simulink model "dual_quaternion_equation_of_motion_2"  (R2016a)
settings: Solver=VariableStepAuto  StartTime=0.0  StopTime=1000  RelTol=1e-3
InitFcn:
  | addpath('..');
libraries: aerolibconvert2 x6
settings Model: Creator=AkhramovichSA  LastModifiedBy=AkhramovichSA

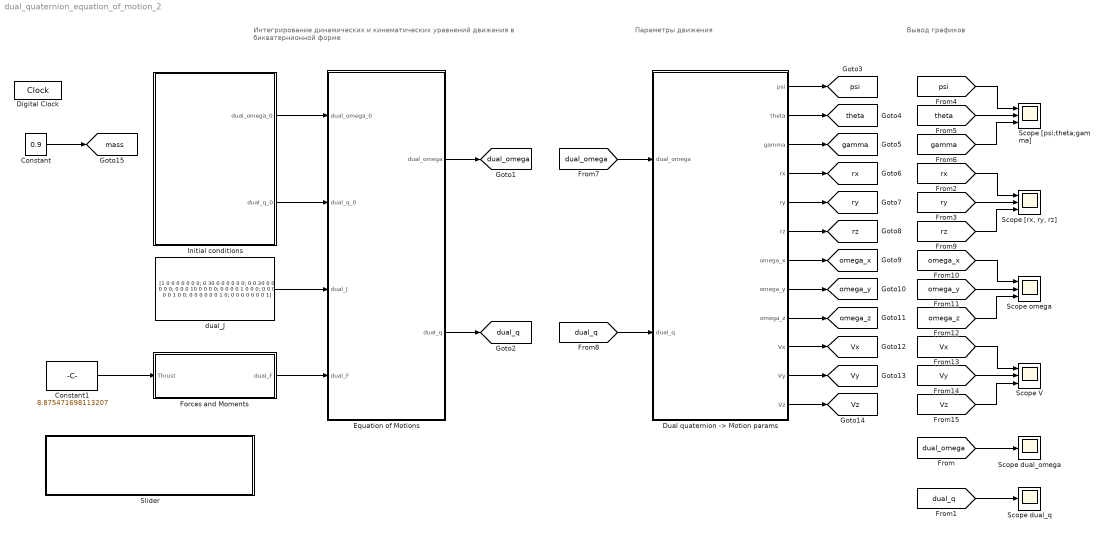
== system dual_quaternion_equation_of_motion_2 ==
  note: Интегрирование динамических и кинематических уравнений движения в бикватернионной форме
  note: Параметры движения
  note: Вывод графиков
  Constant : Constant  Value=0.9
  Constant1 : Constant  Value=8.875471698113207
  Digital Clock : DigitalClock  SampleTime=0.01
  "Dual quaternion -> Motion params" : MATLAB Function  TreatAsAtomicUnit=on
  Equation of Motions : Subsystem
  Forces and Moments : Subsystem
  Initial conditions : Subsystem
  Scope V : Scope  NumInputPorts=3
  Scope [psi;theta;gamma] : Scope  NumInputPorts=3
  "Scope [rx, ry, rz]" : Scope  NumInputPorts=3
  Scope dual_omega : Scope
  Scope dual_q : Scope
  Scope omega : Scope  NumInputPorts=3
  Slider : Subsystem  DialogController=hmiCreateDDGDialog  IsWebBlock=on  mask(MWDashboardBlock){webBlockId=836bae8a-61ff-49e9-8a0b-c22522f8dc87, webBlockType=slider, ShowInLibBrowser=on, ShowInitialText=on, HMISrcModelName=dual_quaternion_equation_of_motion_2}
      mask prompts: webBlockId "WebBlock Id"; webBlockType "WebBlock Type"; HMISrcModelName "Source Model"
      mask Help: helpview([docroot '/mapfiles/simulink.map'], 'hmi_slider')
      mask Display:
      | if strcmp(get_param(bdroot(gcb),'BlockDiagramType'), 'library')
      |     image([(matlabroot) '/toolbox/simulink/hmi/icons/Slider.png']);
      | end
  dual_J : Constant  Value=[1 0 0 0 0 0 0 0; 0 30 0 0 0 0 0 0; 0 0 20 0 0 0 0 0; 0 0 0 10 0 0 0 0; 0 0 0 0 1 0 0 0; 0 0 0 0 0 1 0 0; 0 0 0 0 0 0 1 0; 0 0 0 0 0 0 0 1]  VectorParams1D=off
  tag scope: Vx=global, Vy=global, Vz=global, dual_omega=global, dual_q=global, gamma=global, mass=global, omega_x=global, omega_y=global, omega_z=global, psi=global, rx=global, ry=global, rz=global, theta=global
  wires:
  dual_J/1 -> Equation of Motions/3(dual_J)
  Initial conditions/1(dual_omega_0) -> Equation of Motions/1(dual_omega_0)
  Initial conditions/2(dual_q_0) -> Equation of Motions/2(dual_q_0)
  Forces and Moments/1(dual_F) -> Equation of Motions/4(dual_F)
  Equation of Motions/1(dual_omega) -> [dual_omega]
  [dual_omega] -> Scope dual_omega/1
  Equation of Motions/2(dual_q) -> [dual_q]
  [dual_q] -> Scope dual_q/1
  [psi] -> Scope [psi;theta;gamma]/1
  [theta] -> Scope [psi;theta;gamma]/2
  [gamma] -> Scope [psi;theta;gamma]/3
  [dual_omega] -> "Dual quaternion -> Motion params"/1(dual_omega)
  [dual_q] -> "Dual quaternion -> Motion params"/2(dual_q)
  "Dual quaternion -> Motion params"/1(psi) -> [psi]
  "Dual quaternion -> Motion params"/2(theta) -> [theta]
  "Dual quaternion -> Motion params"/3(gamma) -> [gamma]
  "Dual quaternion -> Motion params"/4(rx) -> [rx]
  "Dual quaternion -> Motion params"/5(ry) -> [ry]
  "Dual quaternion -> Motion params"/6(rz) -> [rz]
  "Dual quaternion -> Motion params"/7(omega_x) -> [omega_x]
  "Dual quaternion -> Motion params"/9(omega_z) -> [omega_z]
  "Dual quaternion -> Motion params"/8(omega_y) -> [omega_y]
  "Dual quaternion -> Motion params"/10(Vx) -> [Vx]
  "Dual quaternion -> Motion params"/11(Vy) -> [Vy]
  "Dual quaternion -> Motion params"/12(Vz) -> [Vz]
  [rx] -> "Scope [rx, ry, rz]"/1
  [ry] -> "Scope [rx, ry, rz]"/2
  [rz] -> "Scope [rx, ry, rz]"/3
  [omega_x] -> Scope omega/1
  [omega_y] -> Scope omega/2
  [omega_z] -> Scope omega/3
  [Vx] -> Scope V/1
  [Vy] -> Scope V/2
  [Vz] -> Scope V/3
  Constant/1 -> [mass]
  Constant1/1 -> Forces and Moments/1(Thrust)

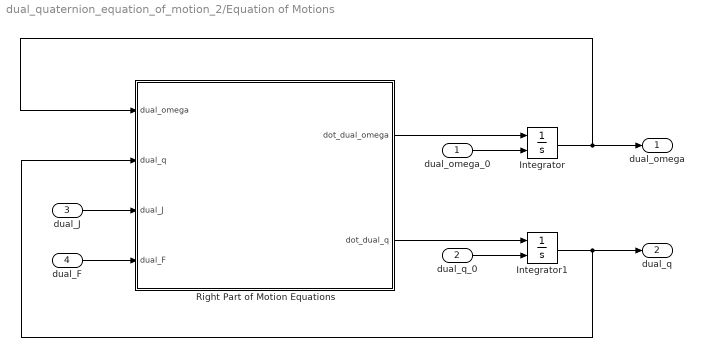
== system dual_quaternion_equation_of_motion_2/Equation of Motions ==
  dual_omega_0 : Inport
  dual_q_0 : Inport  Port=2
  dual_J : Inport  Port=3
  dual_F : Inport  Port=4
  Integrator : Integrator  InitialConditionSource=external
  Integrator1 : Integrator  InitialConditionSource=external
  Right Part of Motion Equations : MATLAB Function  TreatAsAtomicUnit=on
  dual_omega : Outport
  dual_q : Outport  Port=2
  wires:
  Integrator/1 -> dual_omega/1, Right Part of Motion Equations/1(dual_omega)
  dual_omega_0/1 -> Integrator/2
  dual_q_0/1 -> Integrator1/2
  Right Part of Motion Equations/1(dot_dual_omega) -> Integrator/1
  Integrator1/1 -> dual_q/1, Right Part of Motion Equations/2(dual_q)
  Right Part of Motion Equations/2(dot_dual_q) -> Integrator1/1
  dual_F/1 -> Right Part of Motion Equations/4(dual_F)
  dual_J/1 -> Right Part of Motion Equations/3(dual_J)

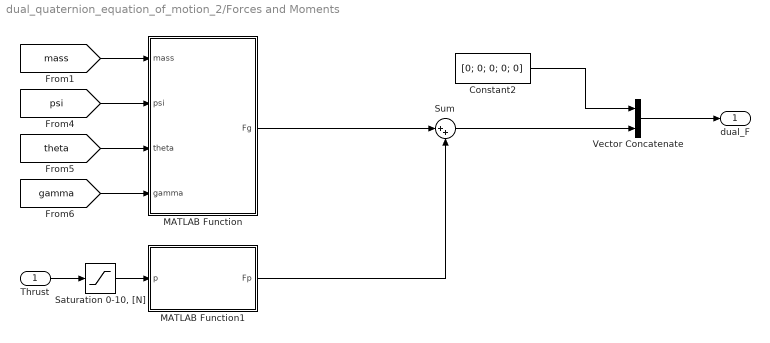
== system dual_quaternion_equation_of_motion_2/Forces and Moments ==
  Thrust : Inport
  Constant2 : Constant  Value=[0; 0; 0; 0; 0]
  MATLAB Function : MATLAB Function  TreatAsAtomicUnit=on
  MATLAB Function1 : MATLAB Function  TreatAsAtomicUnit=on
  "Saturation 0-10, [N]" : Saturate  UpperLimit=10  LowerLimit=0
  Sum : Sum  Inputs=|++
  Vector Concatenate : Concatenate
  dual_F : Outport
  wires:
  [mass] -> MATLAB Function/1(mass)
  [psi] -> MATLAB Function/2(psi)
  [theta] -> MATLAB Function/3(theta)
  [gamma] -> MATLAB Function/4(gamma)
  MATLAB Function1/1(Fp) -> Sum/2
  MATLAB Function/1(Fg) -> Sum/1
  Sum/1 -> Vector Concatenate/2
  Vector Concatenate/1 -> dual_F/1
  Constant2/1 -> Vector Concatenate/1
  Thrust/1 -> "Saturation 0-10, [N]"/1
  "Saturation 0-10, [N]"/1 -> MATLAB Function1/1(p)

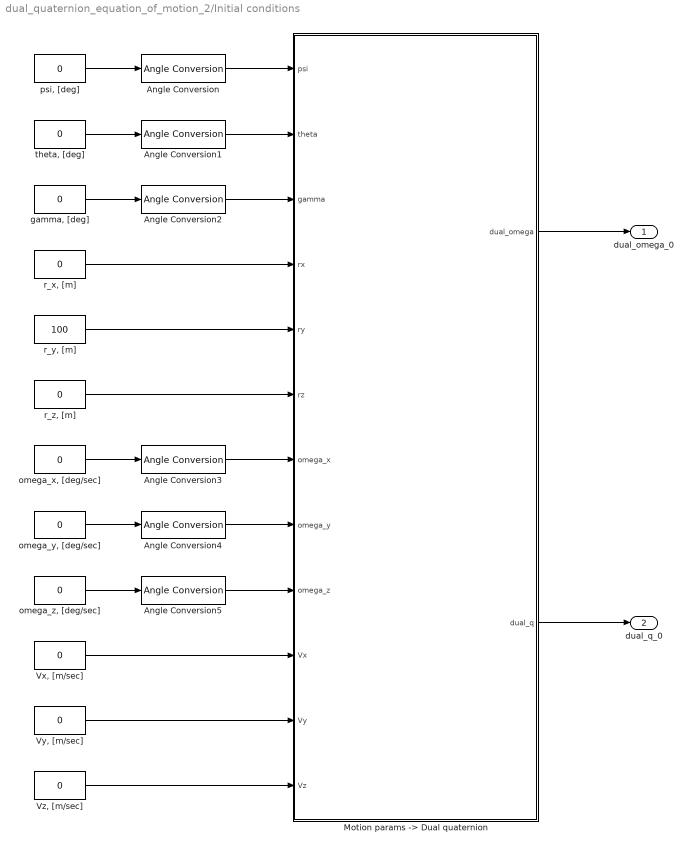
== system dual_quaternion_equation_of_motion_2/Initial conditions ==
  Angle Conversion{,1..5} (6 alike) : aerolibconvert2/Angle Conversion  IU=deg  OU=rad
  "Motion params -> Dual quaternion" : MATLAB Function  TreatAsAtomicUnit=on
  "Vx, [m/sec]" : Constant  Value=0  VectorParams1D=off
  "Vy, [m/sec]" : Constant  Value=0  VectorParams1D=off
  "Vz, [m/sec]" : Constant  Value=0  VectorParams1D=off
  "gamma, [deg]" : Constant  Value=0  VectorParams1D=off
  "omega_x, [deg/sec]" : Constant  Value=0  VectorParams1D=off
  "omega_y, [deg/sec]" : Constant  Value=0  VectorParams1D=off
  "omega_z, [deg/sec]" : Constant  Value=0  VectorParams1D=off
  "psi, [deg]" : Constant  Value=0  VectorParams1D=off
  "r_x, [m]" : Constant  Value=0  VectorParams1D=off
  "r_y, [m]" : Constant  Value=100  VectorParams1D=off
  "r_z, [m]" : Constant  Value=0  VectorParams1D=off
  "theta, [deg]" : Constant  Value=0  VectorParams1D=off
  dual_omega_0 : Outport
  dual_q_0 : Outport  Port=2
  wires:
  "psi, [deg]"/1 -> Angle Conversion/1
  "theta, [deg]"/1 -> Angle Conversion1/1
  "gamma, [deg]"/1 -> Angle Conversion2/1
  "r_x, [m]"/1 -> "Motion params -> Dual quaternion"/4(rx)
  "r_y, [m]"/1 -> "Motion params -> Dual quaternion"/5(ry)
  "r_z, [m]"/1 -> "Motion params -> Dual quaternion"/6(rz)
  "Motion params -> Dual quaternion"/1(dual_omega) -> dual_omega_0/1
  "Motion params -> Dual quaternion"/2(dual_q) -> dual_q_0/1
  "omega_x, [deg/sec]"/1 -> Angle Conversion3/1
  "omega_y, [deg/sec]"/1 -> Angle Conversion4/1
  "omega_z, [deg/sec]"/1 -> Angle Conversion5/1
  "Vx, [m/sec]"/1 -> "Motion params -> Dual quaternion"/10(Vx)
  "Vy, [m/sec]"/1 -> "Motion params -> Dual quaternion"/11(Vy)
  "Vz, [m/sec]"/1 -> "Motion params -> Dual quaternion"/12(Vz)
  Angle Conversion/1 -> "Motion params -> Dual quaternion"/1(psi)
  Angle Conversion1/1 -> "Motion params -> Dual quaternion"/2(theta)
  Angle Conversion2/1 -> "Motion params -> Dual quaternion"/3(gamma)
  Angle Conversion3/1 -> "Motion params -> Dual quaternion"/7(omega_x)
  Angle Conversion4/1 -> "Motion params -> Dual quaternion"/8(omega_y)
  Angle Conversion5/1 -> "Motion params -> Dual quaternion"/9(omega_z)

== system dual_quaternion_equation_of_motion_2/Slider ==

== matlab function dual_quaternion_equation_of_motion_2/Initial conditions/Motion params -> Dual quaternion ==
  data: psi input; dual_omega output; dual_q output; theta input; gamma input; rx input; ry input; rz input; omega_x input; omega_y input; omega_z input; Vx input; Vy input; Vz input
function [dual_omega, dual_q] = motion_params_to_dual_quaternion(psi, theta, gamma, rx, ry, rz, omega_x, omega_y, omega_z, Vx, Vy, Vz)
% Перевод параметров движения в бикватернионную форму

coder.extrinsic('dq_from_euler_translation'); % for simulink

dual_q     = [1; zeros(7, 1)];

dual_omega = [0; omega_x; omega_y; omega_z;  0; Vx; Vy; Vz];  % Начальная углоавя и линейная скорости
dual_q     = dq_from_euler_translation([psi; theta; gamma], [rx; ry; rz]);      % Начальное ориентация и положение ЛА

== matlab function dual_quaternion_equation_of_motion_2/Equation of Motions/Right Part of Motion Equations ==
  data: dual_omega input; dot_dual_omega output; dual_q input; dual_J input; dot_dual_q output; dual_F input
function [dot_dual_omega, dot_dual_q] = dot_dual_omega_q(dual_omega, dual_q, dual_J, dual_F)
% Правые части динамического и кинематического уравнений движения в бикватернионной форме
% Выходные данные надо проинтегрировать звеном: 1/s

% Входные данные:
%
% Бикватернион угловых и линейных скоростей
% dual_omega = [0; omega_x; omega_y; omega_z; 0; v_x; v_y; v_z]
%
% Бикватернион углового и линейного положения
% dual_q     = [q1; q2; q3; q4; q5; q6; q7; q8]
% 
% Бикватернион моментов и сил
% dual_F     = [0; Mx; My; Mz; 0; Fx; Fy; Fz]
%
% Расширенный тензор инерции в бикватернионной форме
% dual_J     = [1  0   0   0  0  0  0  0;
%               0 Jxx Jxy Jxz 0  0  0  0;
%               0 Jyx Jyy Jyz 0  0  0  0;
%               0 Jzx Jzy Jzz 0  0  0  0;
%               0  0   0   0  1  0  0  0;
%               0  0   0   0  0  m  0  0;
%               0  0   0   0  0  0  m  0;
%               0  0   0   0  0  0  0  m]
% 
% Выходные данные:
% 
% Правая часть дифференциального уравнения динамики, изменение бикватерниона угловых и линейных скоростей
% dot_dual_omega = [0; omega_x; omega_y; omega_z; 0; v_x; v_y; v_z]
%
% Правая часть дифференциального уравнения кинематики, изменение бикватерниона углового и линейного положения
% dot_dual_q     = [q1; q2; q3; q4; q5; q6; q7; q8]

dot_dual_omega = dual_J \ (dual_F - dq_cross([dual_omega(1:4); 0; 0; 0; 0], (dual_J*dual_omega))); 

dot_dual_q     = 0.5*dq_multiply(dual_q, dual_omega);

== matlab function dual_quaternion_equation_of_motion_2/Forces and Moments/MATLAB Function ==
  data: mass input; Fg output; psi input; theta input; gamma input
function Fg = force_gravity(mass, psi, theta, gamma)

Fg_nsk = [0; -9.81*mass; 0];

Fg     = nsk2ssk(gamma, psi, theta)*Fg_nsk;

== matlab function dual_quaternion_equation_of_motion_2/Forces and Moments/MATLAB Function1 ==
  data: p input; Fp output
function Fp = force_thrust(p)

Fp = [0; p; 0];

== matlab function dual_quaternion_equation_of_motion_2/Dual quaternion -> Motion params ==
  data: dual_omega input; psi output; theta output; dual_q input; gamma output; rx output; ry output; rz output; omega_x output; omega_y output; omega_z output; Vx output; Vy output; Vz output
function [psi, theta, gamma, rx, ry, rz, omega_x, omega_y, omega_z, Vx, Vy, Vz] = dual_quaternion_to_motion_params(dual_omega, dual_q)
% Перевод в бикватернионна скорости и положения в параметры движения

coder.extrinsic('dq_get_rotation_euler', 'dq_get_translation_vector'); % for simulink

omega   = dual_omega(2:4); % Угловая скорость, [рад/с]
omega_x = omega(1);
omega_y = omega(2);
omega_z = omega(3);

V  = dual_omega(6:8); % Линейная скорость, [м/с]
Vx = V(1);
Vy = V(2);
Vz = V(3);

psi   = 0;
theta = 0;
gamma = 0;
[psi, theta, gamma] = dq_get_rotation_euler(dual_q);     % Углы ориентации, [рад]

r  = zeros(3,1);
r  = dq_get_translation_vector(dual_q); % Радиус-вектор положения ЛА, [м]
rx = r(1);
ry = r(2);
rz = r(3);
